simulink model "Assignment_II_4"  (Simulink 8.6)
settings: Solver=ode1  StartTime=0.0  StopTime=10  FixedStep=1/5000  RelTol=1e-3
PostLoadFcn:
  | , if any(exist('dsrtsu_mdlpostloadfcn', 'file') == [2, 3, 6]), try dsrtsu_mdlpostloadfcn('Execute', bdroot); catch fprintf('Error in PostLoadFcn (dsrtsu_mdlpostloadfcn) for model "%s":\n %s\n', bdroot, lasterr); end, end,
values from neighbouring files (symbols this model uses):
  C_den = 1    [assignment4.m]
  C_num = num    [assignment4.m]
  I0 = 2.36    [Assignment3.mat]    (also in assignment3.m = I(2))
  Y0 = 0.049    [Assignment3.mat]    (also in assignment3.m = Y(2))
undefined symbols (not defined in the file or in its folder): P_den, P_num
settings Model: DSRTSU_INTERNAL_RTI_VER=350  DSRTSU_INTERNAL_RTI_TYPE=rti1104  Creator=kverkerk  LastModifiedBy=s127283
settings OptimizationCC: BlockReduction=off  OptimizeBlockIOStorage=off  BufferReuse=off  GlobalBufferReuse=off  ExpressionFolding=off  LocalBlockOutputs=off
settings DebuggingCC: FcnCallInpInsideContextMsg=UseLocalSettings
settings HardwareCC: ProdIntDivRoundTo=Zero  ProdEndianess=BigEndian  ProdHWDeviceType=Generic->Custom  TargetIntDivRoundTo=Zero  TargetEndianess=BigEndian  TargetHWDeviceType=Generic->Custom
settings RTWCC: SystemTargetFile=rti1104.tlc  MakeCommand=make_rti  TemplateMakefile=rti1104.tmf  Description=dSPACE DS1104 Hardware Platform
settings STFCustomTargetCC: MatFileLogging=on  CPPClassGenCompliant=on  SystemTargetFile=rti1104.tlc
settings GRTTargetCC: ParMdlRefBuildCompliant=off  CompOptLevelCompliant=off  ConcurrentExecutionCompliant=off  GeneratePreprocessorConditionals=Use local settings  UseToolchainInfoCompliant=off  ExtModeMexFile=noextcomm
settings CustomProperty: DataType=RTWOptions_EnumType_C__dSPACE6p5_matlab_rti1104_tlc_rti1104_1InitialSimState  Value=RUN
settings EnumStrPairs: String=RUN

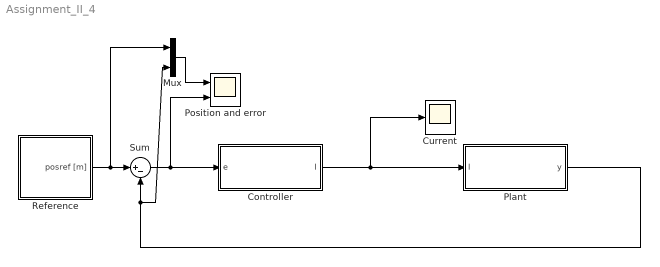
== system Assignment_II_4 ==
  Controller : Subsystem
  Current : Scope
  Mux : Mux  Inputs=2
  Plant : Subsystem
  Position and error : Scope  NumInputPorts=2
  Reference : Subsystem
  Sum : Sum  Inputs=|+-
  wires:
  Controller/1(I) -> Plant/1(I), Current/1
  Reference/1(posref [m]) -> Sum/1, Mux/1
  Sum/1 -> Position and error/2, Controller/1(e)
  Plant/1(y) -> Sum/2, Mux/2
  Mux/1 -> Position and error/1

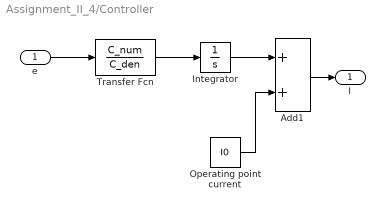
== system Assignment_II_4/Controller ==
  e : Inport
  Add1 : Sum
  Integrator : Integrator  LimitOutput=on  UpperSaturationLimit=3-I0  LowerSaturationLimit=-I0
  Operating point current : Constant  Value=I0
  Transfer Fcn : TransferFcn  Numerator=C_num  Denominator=C_den
  I : Outport
  wires:
  e/1 -> Transfer Fcn/1
  Operating point current/1 -> Add1/2
  Add1/1 -> I/1
  Transfer Fcn/1 -> Integrator/1
  Integrator/1 -> Add1/1

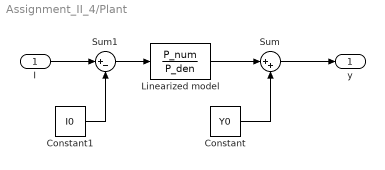
== system Assignment_II_4/Plant ==
  I : Inport
  Constant : Constant  Value=Y0
  Constant1 : Constant  Value=I0
  Linearized model : TransferFcn  Numerator=P_num  Denominator=P_den
  Sum : Sum  Inputs=|++
  Sum1 : Sum  Inputs=|+-
  y : Outport
  wires:
  Linearized model/1 -> Sum/1
  Sum/1 -> y/1
  Constant/1 -> Sum/2
  Sum1/1 -> Linearized model/1
  Constant1/1 -> Sum1/2
  I/1 -> Sum1/1

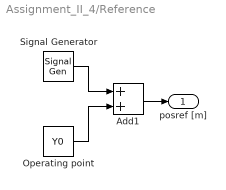
== system Assignment_II_4/Reference ==
  Add1 : Sum
  Operating point : Constant  Value=Y0
  Signal Generator : SignalGenerator  Amplitude=1e-3
  posref [m] : Outport
  wires:
  Signal Generator/1 -> Add1/1
  Add1/1 -> posref [m]/1
  Operating point/1 -> Add1/2
